simulink model "sim_validation_6DoF"  (R2025a)
settings: Solver=VariableStepAuto  StartTime=0.0  StopTime=tf  RelTol=1e-12  AbsTol=1e-12
values from neighbouring files (symbols this model uses):
  alpha = 0.5086    [3DoF_deterministic_Workspace.mat]    (also in Compressed_Time_Step_2dof_Experiment.mat; Copy_of_Deterministic_6DoF.m; Copy_of_Deterministic_6DoF_quat.m; Copy_of_SCP_Earth_Mars_transfer_GA_uniform_adaptive.m = 1)
  I = 0.15    [3DoF_deterministic_Workspace.mat]    (also in Copy_of_DQG_6DoF_fixedtf.m = [4.2; 4.2; 0.6]; Copy_of_Deterministic_6DoF.m = [50000; 150000; 150000] * (1e-3) ^ 2; Copy_of_Deterministic_6DoF_quat.m = [50000; 150000; 150000] * (1e-3) ^ 2; DQG_6DoF.m = [4.2; 4.2; 0.6])
  I_matrix = diag([I/5, I, I])    [Deterministic_3DoF_with_mass_convexified_reynolds.m]    (also in Deterministic_3DoF_with_mass_convexified_takeoffdivert.m; Deterministic_6DoF_reynolds.m = diag(I); Deterministic_6DoF_reynolds_quat.m = diag(I); Deterministic_6DoF_reynolds_quat_alphabeta.m = diag(I))
  input_vector = 1:nu    [Deterministic_3DoF_with_mass_convexified_reynolds.m]    (also in Deterministic_3DoF_with_mass_convexified_takeoffdivert.m; Deterministic_3DoF_with_mass_polar.m; Deterministic_6DoF_reynolds.m; Deterministic_6DoF_reynolds_quat.m)
  L = 0.003    [3DoF_deterministic_Workspace.mat]    (also in Compressed_Time_Step_2dof_Experiment.mat; Copy_of_DQG_6DoF_fixedtf.m = 1; Copy_of_Deterministic_6DoF.m; Copy_of_Deterministic_6DoF_quat.m)
  m_0 = 2100    [3DoF_deterministic_Workspace.mat]    (also in Compressed_Time_Step_2dof_Experiment.mat = 2000; Copy_of_Deterministic_6DoF.m = 2600; Copy_of_Deterministic_6DoF_quat.m = 2600; Copy_of_SCP_Earth_Mars_transfer_GA_uniform_adaptive.m = 1)
  m_dry = 1500    [3DoF_deterministic_Workspace.mat]    (also in Copy_of_Deterministic_6DoF.m = 2000; Copy_of_Deterministic_6DoF_quat.m = 2000; Deterministic_3DoF.m = 2000; Deterministic_3DoF_with_mass.m)
  m_wet = 600    [3DoF_deterministic_Workspace.mat]    (also in Copy_of_Deterministic_6DoF.m; Copy_of_Deterministic_6DoF_quat.m; Deterministic_3DoF.m; Deterministic_3DoF_with_mass.m)
  r_0_6DoF = [r_0(1); 0; r_0(2)]    [Deterministic_3DoF_with_mass_convexified_reynolds.m]    (also in Deterministic_3DoF_with_mass_convexified_takeoffdivert.m; Deterministic_6DoF_reynolds.m = r_0; Deterministic_6DoF_reynolds_quat.m = r_0; Deterministic_6DoF_reynolds_quat_alphabeta.m = r_0)
  v_0_b_6DoF = [v_0_b(1); 0; v_0_b(2)]    [Deterministic_3DoF_with_mass_convexified_reynolds.m]    (also in Deterministic_3DoF_with_mass_convexified_takeoffdivert.m; Deterministic_6DoF_reynolds.m = v_0_b; Deterministic_6DoF_reynolds_quat.m = quat_rot(q_conj(q_0), v_0); Deterministic_6DoF_reynolds_quat_alphabeta.m = quat_rot(q_conj(q_0), v_0))
  x_0_6DoF = [r_0_6DoF; v_0_6DoF; rpy_0_6DoF; w_0_6DoF; log(m_0)]    [Deterministic_3DoF_with_mass_convexified_reynolds.m]    (also in Deterministic_3DoF_with_mass_convexified_takeoffdivert.m; Deterministic_6DoF_reynolds.m = [r_0_6DoF; v_0_6DoF; rpy_0_6DoF; w_0_6DoF]; Deterministic_6DoF_reynolds_quat.m = x_0; Deterministic_6DoF_reynolds_quat_alphabeta.m = x_0)
libraries: simulink_extras x2, aerolibanim x1, aerolibobsolete x1
settings Model: Creator=thatf  LastModifiedBy=thatf

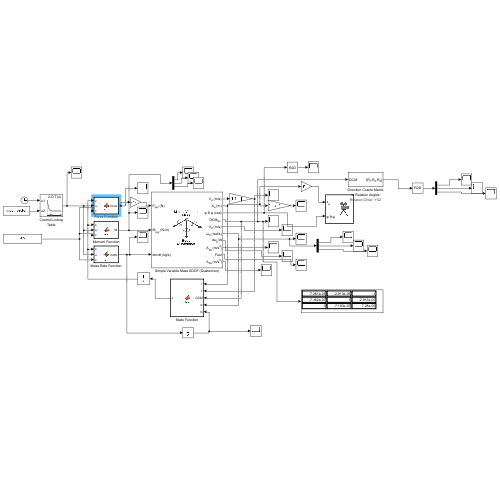
[thumbnail: Simulink's stored preview of the top-level diagram]
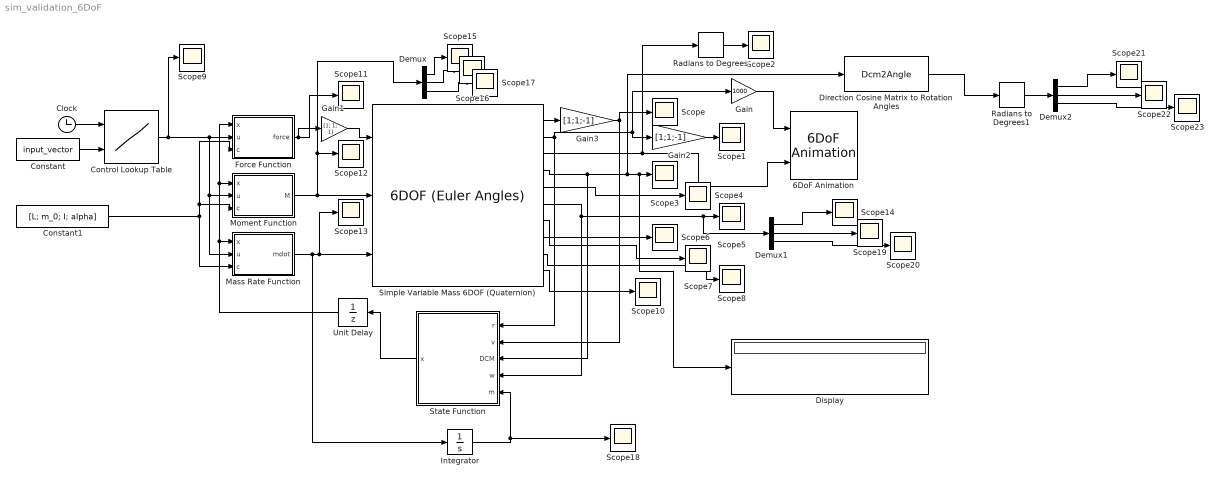
== system sim_validation_6DoF ==
  6DoF Animation : aerolibanim/6DoF Animation  u1=[-1000 1000 -100 100 -5000 50]  u2=0.1  u3=100  u4=[0 0 0]  u5=Fly alongside  u6=[0 1000 0]  u7=80  u8=off
  Clock : Clock
  Constant : Constant  Value=input_vector
  Constant1 : Constant  Value=[L; m_0; I; alpha]
  Control Lookup Table : Lookup_n-D  BreakpointsForDimension1=opt_time'  BreakpointsForDimension2=input_vector  Table=control_inputs'  InternalRulePriority=Speed  RndMeth=Simplest
      settings: InputPortMap=u0,u1
  Demux : Demux  Outputs=3
  Demux1 : Demux  Outputs=3
  Demux2 : Demux  Outputs=3
  Direction Cosine Matrix to Rotation Angles : Dcm2Angle  rotationOrder=YXZ
      settings: AttributesFormatString=Rotation Order: %<rotationOrder>
  Display : Display
  Force Function : MATLAB Function  TreatAsAtomicUnit=on
  Gain : Gain  Gain=1000
  Gain1 : Gain  Gain=[1; 1; 1]
  Gain2 : Gain  Gain=[1;1;-1]
  Gain3 : Gain  Gain=[1;1;-1]
  Integrator : Integrator  InitialCondition=m_0
  Mass Rate Function : MATLAB Function  TreatAsAtomicUnit=on
  Moment Function : MATLAB Function  TreatAsAtomicUnit=on
  Radians to Degrees : simulink_extras/Transformations/Radians to Degrees
  Radians to Degrees1 : simulink_extras/Transformations/Radians to Degrees
  Scope{,1..23} (24 alike) : Scope
      Scope settings: ActiveDisplayYMinimum=-0.05945416991082874  ActiveDisplayYMaximum=0.18508752919745861
      Scope1 settings: ActiveDisplayYMinimum=-0.032533542912153809  ActiveDisplayYMaximum=0.77268972882108777
      Scope10 settings: ActiveDisplayYMinimum=-1  ActiveDisplayYMaximum=1  DataLoggingVariableName=ScopeData2
      Scope11 settings: ActiveDisplayYMinimum=-9.19206  ActiveDisplayYMaximum=14.49525
      Scope12 settings: ActiveDisplayYMinimum=-0.00032954774637783732  ActiveDisplayYMaximum=0.00046685662694902842  DataLoggingVariableName=ScopeData2
      Scope13 settings: ActiveDisplayYMinimum=-1  ActiveDisplayYMaximum=1  DataLoggingVariableName=ScopeData3
      Scope14 settings: ActiveDisplayYMinimum=-0.42348452135333808  ActiveDisplayYMaximum=0.42087304065501741  DataLoggingVariableName=ScopeData9
      Scope15 settings: ActiveDisplayYMinimum=0.08257  ActiveDisplayYMaximum=0.10257  DataLoggingVariableName=ScopeData2
      Scope16 settings: ActiveDisplayYMinimum=-1  ActiveDisplayYMaximum=1  DataLoggingVariableName=ScopeData3
      Scope17 settings: ActiveDisplayYMinimum=-1  ActiveDisplayYMaximum=1  DataLoggingVariableName=ScopeData4
      Scope18 settings: ActiveDisplayYMinimum=3078.5395308444149  ActiveDisplayYMaximum=3129.985756084528  DataLoggingVariableName=ScopeData5
      Scope19 settings: ActiveDisplayYMinimum=-0.42348452135333808  ActiveDisplayYMaximum=0.42087304065501741  DataLoggingVariableName=ScopeData10
      Scope2 settings: ActiveDisplayYMinimum=-273.77709634457119  ActiveDisplayYMaximum=289.05644106186958  DataLoggingVariableName=ScopeData2
      Scope20 settings: ActiveDisplayYMinimum=-0.42348452135333808  ActiveDisplayYMaximum=0.42087304065501741  DataLoggingVariableName=ScopeData11
      Scope21 settings: ActiveDisplayYMinimum=53.1292524959417  ActiveDisplayYMaximum=144.41382609165456  DataLoggingVariableName=ScopeData12
      Scope22 settings: ActiveDisplayYMinimum=-2.0266782779062082  ActiveDisplayYMaximum=0.22518647532291197  DataLoggingVariableName=ScopeData13
      Scope23 settings: ActiveDisplayYMinimum=-4.92871242540069  ActiveDisplayYMaximum=3.4395423986524243  DataLoggingVariableName=ScopeData14
      Scope3 settings: ActiveDisplayYMinimum=-1  ActiveDisplayYMaximum=1  DataLoggingVariableName=ScopeData3
      Scope4 settings: ActiveDisplayYMinimum=-0.049785628433832184  ActiveDisplayYMaximum=0.14529640553378664  DataLoggingVariableName=ScopeData4
      Scope5 settings: ActiveDisplayYMinimum=-0.42348452135333808  ActiveDisplayYMaximum=0.42087304065501741  DataLoggingVariableName=ScopeData5
      Scope6 settings: ActiveDisplayYMinimum=-1  ActiveDisplayYMaximum=1  DataLoggingVariableName=ScopeData6
      Scope7 settings: ActiveDisplayYMinimum=-1  ActiveDisplayYMaximum=1  DataLoggingVariableName=ScopeData7
      Scope8 settings: ActiveDisplayYMinimum=-1  ActiveDisplayYMaximum=1  DataLoggingVariableName=ScopeData8
      Scope9 settings: ActiveDisplayYMinimum=-1  ActiveDisplayYMaximum=1
  Simple Variable Mass 6DOF (Quaternion) : aerolibobsolete/6DOF (Euler Angles)  units=Metric (MKS)  mtype=Simple Variable  rep=Quaternion  xme_0=r_0_6DoF .* [1;1;-1]  Vm_0=v_0_b_6DoF .* [1;1;-1]  eul_0=rpy_0_6DoF  pm_0=w_0_6DoF  mass_0=m_0  mass_e=m_dry  mass_f=m_wet + m_dry  inertia=eye(3)  inertia_e=I_matrix - 1e-12  inertia_f=I_matrix  k_quat=1.0  vre_flag=off  abi_flag=on  aMode=0  xme_statename=''  Vm_statename=''  eul_statename=''  quat_statename=''  pm_statename=''  mass_statename=''
  State Function : MATLAB Function  TreatAsAtomicUnit=on
  Unit Delay : UnitDelay  InitialCondition=x_0_6DoF  SampleTime=-1  HasFrameUpgradeWarning=on
  wires:
  Force Function/1(force) -> Gain1/1, Scope11/1
  Moment Function/1(M) -> Demux/1, Scope12/1, Simple Variable Mass 6DOF (Quaternion)/2
  Mass Rate Function/1(mdot) -> Integrator/1, Simple Variable Mass 6DOF (Quaternion)/3, Scope13/1
  Simple Variable Mass 6DOF (Quaternion)/3 -> 6DoF Animation/2, Radians to Degrees/1
  Simple Variable Mass 6DOF (Quaternion)/4 -> State Function/3(DCM), Direction Cosine Matrix to Rotation Angles/1, Display/1, Scope3/1
  Simple Variable Mass 6DOF (Quaternion)/5 -> Scope4/1
  Simple Variable Mass 6DOF (Quaternion)/6 -> State Function/4(w), Demux1/1, Scope5/1
  Simple Variable Mass 6DOF (Quaternion)/7 -> Scope6/1
  Simple Variable Mass 6DOF (Quaternion)/8 -> Scope7/1
  Simple Variable Mass 6DOF (Quaternion)/9 -> Scope8/1
  Simple Variable Mass 6DOF (Quaternion)/2 -> Gain2/1, Gain/1, State Function/1(r)
  Constant1/1 -> Moment Function/3(c), Force Function/3(c), Mass Rate Function/3(c)
  Constant/1 -> Control Lookup Table/2
  Clock/1 -> Control Lookup Table/1
  Control Lookup Table/1 -> Scope9/1, Force Function/2(u), Mass Rate Function/2(u), Moment Function/2(u)
  Integrator/1 -> State Function/5(m), Scope18/1
  Simple Variable Mass 6DOF (Quaternion)/10 -> Scope10/1
  Gain/1 -> 6DoF Animation/1
  State Function/1(x) -> Unit Delay/1
  Demux/2 -> Scope16/1
  Demux/1 -> Scope15/1
  Demux/3 -> Scope17/1
  Radians to Degrees/1 -> Scope2/1
  Gain1/1 -> Simple Variable Mass 6DOF (Quaternion)/1
  Gain2/1 -> Scope1/1
  Simple Variable Mass 6DOF (Quaternion)/1 -> Gain3/1
  Gain3/1 -> State Function/2(v), Scope/1
  Unit Delay/1 -> Force Function/1(x), Moment Function/1(x), Mass Rate Function/1(x)
  Demux1/1 -> Scope14/1
  Demux1/2 -> Scope19/1
  Demux1/3 -> Scope20/1
  Demux2/2 -> Scope22/1
  Demux2/1 -> Scope21/1
  Direction Cosine Matrix to Rotation Angles/1 -> Radians to Degrees1/1
  Demux2/3 -> Scope23/1
  Radians to Degrees1/1 -> Demux2/1

== matlab function sim_validation_6DoF/Moment Function ==
  data: x input; u input; M output; c input
function M = fcn(x, u, c)

T = u(1:3);
tau = u(4);
L = c(1);

M = tau .* [1; 0; 0] + cross([-L; 0; 0], T);

== matlab function sim_validation_6DoF/Force Function ==
  data: x input; u input; force output; c input
function force = fcn(x, u, c)
q = x(7:10);
m = x(14);
T = u(1:3);

g = 1.62e-3;

force = T*0 + quat_rot(q_conj(q), [0; 0; g] * m);

== matlab function sim_validation_6DoF/Mass Rate Function ==
  data: x input; u input; mdot output; c input
function mdot = fcn(x, u, c)

T = norm(u(1:3));
tau = u(4);

alpha = c(6);

mdot = -alpha * T - alpha * sqrt(tau ^ 2);

== matlab function sim_validation_6DoF/State Function ==
  data: r input; x output; v input; DCM input; w input; m input
function x = fcn(r, v, DCM, w, m)

q = qexp(RLog(DCM'));

x = [r; v; q; w; m];

end

function [q] = qexp(tau)
    theta = norm(tau);
    u = tau / theta;
    q = [u * sin(theta / 2); cos(theta / 2)];
end

function [tau] = qLog(q)
    N = size(q, 2);
    for k = 1 : N
        w = q(4, k);
        v = q(1:3, k);
        w = w * sign(w);
        v = v * sign(w);
        tau(:, k) = 2 * v * atan2(norm(v), w) / norm(v);
    end
end

function [tau] = RLog(R)
    theta = acos((trace(R) - 1) / 2);
    u = vee(R - R') / (2 * sin(theta));

    tau = theta * u;

    function [tau] = vee(tau_hat)
        tau = [tau_hat(3, 2); tau_hat(1, 3); tau_hat(2, 1)];
    end
end
